simulink model "predador_presa"  (R2015b)
settings: Solver=VariableStepAuto  StartTime=0.0  StopTime=20.0  RelTol=1e-3
values from neighbouring files (symbols this model uses):
  alpha1 = 1.4    [Lab1.m]    (also in MVAD.m)
  alpha2 = 0.7047    [Lab1.m]    (also in MVAD.m = x(2))
  delta1 = 3.1    [Lab1.m]    (also in MVAD.m)
  delta2 = -1.5    [Lab1.m]    (also in MVAD.m)
  N1_inicial = 4    [Lab1.m]    (also in MVAD.m)
  N2_inicial = 1.6144    [Lab1.m]    (also in MVAD.m = x(1))
settings Model: Creator=Alice  LastModifiedBy=Alice

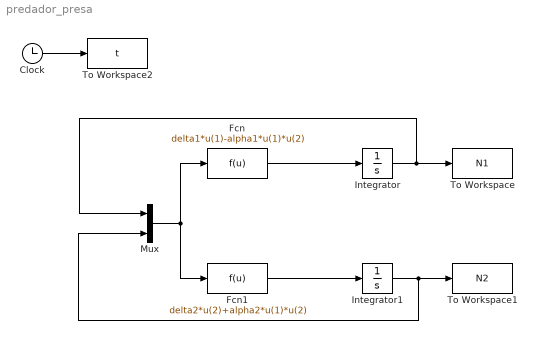
== system predador_presa ==
  Clock : Clock
      settings: Decimation=tt
  Fcn : Fcn  Expr=delta1*u(1)-alpha1*u(1)*u(2)
  Fcn1 : Fcn  Expr=delta2*u(2)+alpha2*u(1)*u(2)
  Integrator : Integrator  InitialCondition=N1_inicial
  Integrator1 : Integrator  InitialCondition=N2_inicial
  Mux : Mux  Inputs=2
  To Workspace : ToWorkspace  VariableName=N1  SampleTime=0.1
  To Workspace1 : ToWorkspace  VariableName=N2  SampleTime=0.1
  To Workspace2 : ToWorkspace  VariableName=t  SampleTime=0.1
  wires:
  Clock/1 -> To Workspace2/1
  Mux/1 -> Fcn/1, Fcn1/1
  Fcn1/1 -> Integrator1/1
  Fcn/1 -> Integrator/1
  Integrator/1 -> Mux/1, To Workspace/1
  Integrator1/1 -> Mux/2, To Workspace1/1
